simulink model "signal_simulation_test"  (R2013a)
settings: Solver=ode3  StartTime=0.0  StopTime=5  FixedStep=0.001  RelTol=1e-3
undefined symbols (not defined in the file or in its folder): sigbuilder_block
settings Model: Creator=Matthias  LastModifiedBy=Matthias

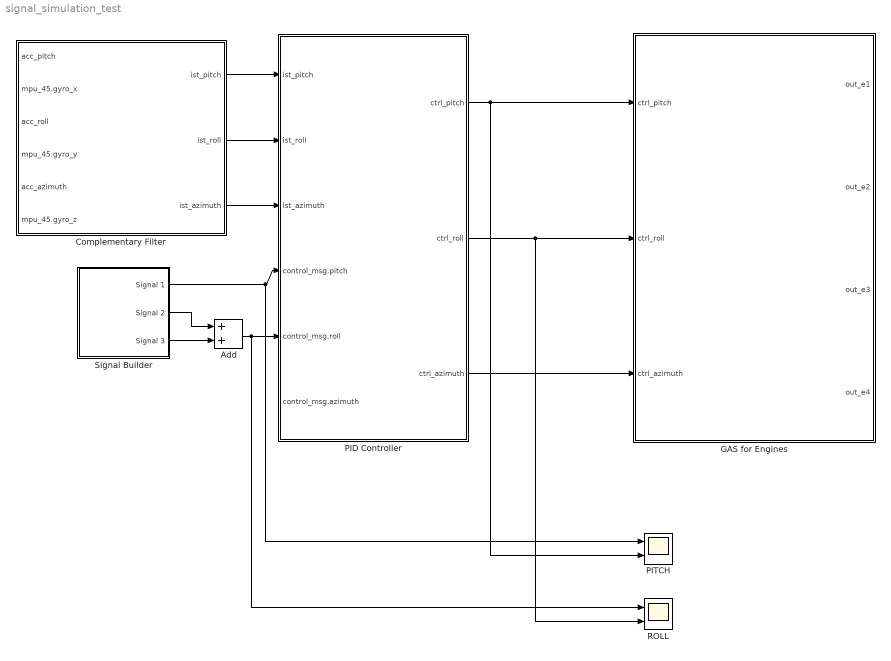
== system signal_simulation_test ==
  Add : Sum
  Complementary Filter : Subsystem
  GAS for Engines : Subsystem
  PID Controller : Subsystem
  PITCH : Scope  NumInputPorts=2
      settings: YMin=-5~-5  YMax=5~5
  ROLL : Scope  NumInputPorts=2
      settings: YMin=-5~-5  YMax=5~5
  Signal Builder : Subsystem  Tag=STV Subsys  LoadFcn=sigbuilder_block('load');  StartFcn=sigbuilder_block('start');  StopFcn=sigbuilder_block('stop');  ClipboardFcn=sigbuilder_block('clipboard');  mask(Sigbuilder block){}
      mask help: Simulink:masks:SigbuilderBlock_MD
      mask init:
      | if ~strcmp(get_param(bdroot(gcbh),'SimulationStatus'),'stopped') tuvar = sigbuilder_block('maskInit'); end
      settings: CopyFcn=sigbuilder_block('copy');  DeleteFcn=sigbuilder_block('delete');  ModelCloseFcn=sigbuilder_block('modelClose');  PreSaveFcn=sigbuilder_block('preSave');  PauseFcn=sigbuilder_block('pause');  ContinueFcn=sigbuilder_block('continue');  NameChangeFcn=sigbuilder_block('namechange');  OpenFcn=sigbuilder_block('open',[437.25 118.5 550.5 394.5 ]);  CloseFcn=sigbuilder_block('close');
      mask Display: plot(0, 0, 100, 100,[2, 2, 32, 32, 2], [68, 8, 8, 68, 68],[32, 2], [38, 38], [32, 19, 2],[53, 60, 44], [32, 17, 17, 2],[16, 16, 31, 31]);txt = getActiveGroup(gcbh);text(2, 100, txt,'verticalAlignment', 'top');
  wires:
  Complementary Filter/1(ist_pitch) -> PID Controller/1(ist_pitch)
  Complementary Filter/2(ist_roll) -> PID Controller/2(ist_roll)
  Complementary Filter/3(ist_azimuth) -> PID Controller/3(ist_azimuth)
  PID Controller/1(ctrl_pitch) -> PITCH/2, GAS for Engines/1(ctrl_pitch)
  PID Controller/2(ctrl_roll) -> ROLL/2, GAS for Engines/2(ctrl_roll)
  PID Controller/3(ctrl_azimuth) -> GAS for Engines/3(ctrl_azimuth)
  Signal Builder/1(Signal 1) -> PITCH/1, PID Controller/4(control_msg.pitch)
  Signal Builder/2(Signal 2) -> Add/1
  Add/1 -> ROLL/1, PID Controller/5(control_msg.roll)
  Signal Builder/3(Signal 3) -> Add/2

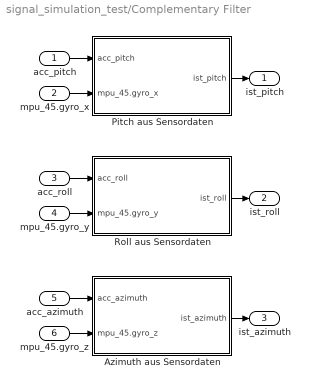
== system signal_simulation_test/Complementary Filter ==
  acc_pitch : Inport
  mpu_45.gyro_x : Inport  Port=2
  acc_roll : Inport  Port=3
  mpu_45.gyro_y : Inport  Port=4
  acc_azimuth : Inport  Port=5
  mpu_45.gyro_z : Inport  Port=6
  Azimuth aus Sensordaten : Subsystem
  Pitch aus Sensordaten : Subsystem
  Roll aus Sensordaten : Subsystem
  ist_pitch : Outport
  ist_roll : Outport  Port=2
  ist_azimuth : Outport  Port=3
  wires:
  acc_pitch/1 -> Pitch aus Sensordaten/1(acc_pitch)
  mpu_45.gyro_x/1 -> Pitch aus Sensordaten/2(mpu_45.gyro_x)
  Roll aus Sensordaten/1(ist_roll) -> ist_roll/1
  Azimuth aus Sensordaten/1(ist_azimuth) -> ist_azimuth/1
  Pitch aus Sensordaten/1(ist_pitch) -> ist_pitch/1
  mpu_45.gyro_y/1 -> Roll aus Sensordaten/2(mpu_45.gyro_y)
  acc_roll/1 -> Roll aus Sensordaten/1(acc_roll)
  mpu_45.gyro_z/1 -> Azimuth aus Sensordaten/2(mpu_45.gyro_z)
  acc_azimuth/1 -> Azimuth aus Sensordaten/1(acc_azimuth)

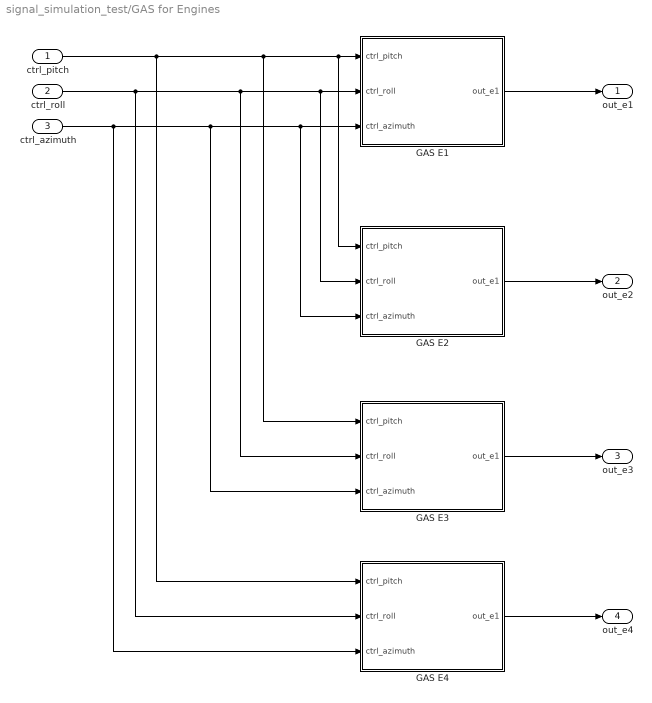
== system signal_simulation_test/GAS for Engines ==
  ctrl_pitch : Inport
  ctrl_roll : Inport  Port=2
  ctrl_azimuth : Inport  Port=3
  GAS E1 : Subsystem
  GAS E2 : Subsystem
  GAS E3 : Subsystem
  GAS E4 : Subsystem
  out_e1 : Outport
  out_e2 : Outport  Port=2
  out_e3 : Outport  Port=3
  out_e4 : Outport  Port=4
  wires:
  ctrl_pitch/1 -> GAS E2/1(ctrl_pitch), GAS E1/1(ctrl_pitch), GAS E3/1(ctrl_pitch), GAS E4/1(ctrl_pitch)
  GAS E1/1(out_e1) -> out_e1/1
  GAS E2/1(out_e1) -> out_e2/1
  ctrl_roll/1 -> GAS E4/2(ctrl_roll), GAS E1/2(ctrl_roll), GAS E2/2(ctrl_roll), GAS E3/2(ctrl_roll)
  GAS E3/1(out_e1) -> out_e3/1
  ctrl_azimuth/1 -> GAS E4/3(ctrl_azimuth), GAS E1/3(ctrl_azimuth), GAS E2/3(ctrl_azimuth), GAS E3/3(ctrl_azimuth)
  GAS E4/1(out_e1) -> out_e4/1

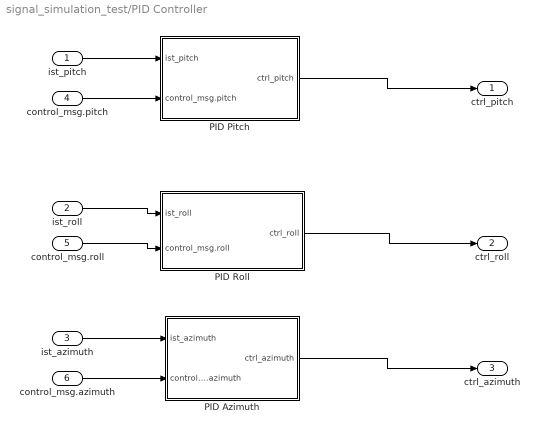
== system signal_simulation_test/PID Controller ==
  ist_pitch : Inport
  ist_roll : Inport  Port=2
  ist_azimuth : Inport  Port=3
  control_msg.pitch : Inport  Port=4
  control_msg.roll : Inport  Port=5
  control_msg.azimuth : Inport  Port=6
  PID Azimuth : Subsystem
  PID Pitch : Subsystem
  PID Roll : Subsystem
  ctrl_pitch : Outport
  ctrl_roll : Outport  Port=2
  ctrl_azimuth : Outport  Port=3
  wires:
  ist_pitch/1 -> PID Pitch/1(ist_pitch)
  control_msg.pitch/1 -> PID Pitch/2(control_msg.pitch)
  ist_azimuth/1 -> PID Azimuth/1(ist_azimuth)
  control_msg.azimuth/1 -> PID Azimuth/2(control_msg.azimuth)
  ist_roll/1 -> PID Roll/1(ist_roll)
  control_msg.roll/1 -> PID Roll/2(control_msg.roll)
  PID Pitch/1(ctrl_pitch) -> ctrl_pitch/1
  PID Roll/1(ctrl_roll) -> ctrl_roll/1
  PID Azimuth/1(ctrl_azimuth) -> ctrl_azimuth/1

== system signal_simulation_test/Signal Builder ==
  Demux : Demux  Tag=STV Demux  Outputs=3
  FromWs : FromWorkspace  Tag=STV FromWs  VariableName=tuvar  SampleTime=0
      SigBuilderData=|
      | common.afterFinalStr = 'Extrapolate'
      | common.sampleTime = 0
      | dataSet.timeRange = [0 10]
      | dataSet.name = 'Group 1'
      | sbobj.Groups.Name = 'Group 1'
      | sbobj.Groups.Signals(1).Name = 'Signal 1'
      | sbobj.Groups.Signals(1).XData = [0 1.02 1.02 3 3 10]
      | sbobj.Groups.Signals(1).YData = [0 0 1 1 0 0]
      | sbobj.Groups.Signals(2).Name = 'Signal 2'
      | sbobj.Groups.Signals(2).XData = [0 3.98 3.98 5.98 5.98 10]
      | sbobj.Groups.Signals(2).YData = [0 0 1 1 0 0]
      | sbobj.Groups.Signals(3).Name = 'Signal 3'
      | sbobj.Groups.Signals(3).XData = [0 7 7 7.96 7.96 10]
      | sbobj.Groups.Signals(3).YData = [0 0 -1.04 -1.04 0 0]
  Signal 1 : Outport  Tag=STV Outport
  Signal 2 : Outport  Tag=STV Outport  Port=2
  Signal 3 : Outport  Tag=STV Outport  Port=3
  wires:
  Demux/1 -> Signal 1/1
  FromWs/1 -> Demux/1
  Demux/2 -> Signal 2/1
  Demux/3 -> Signal 3/1

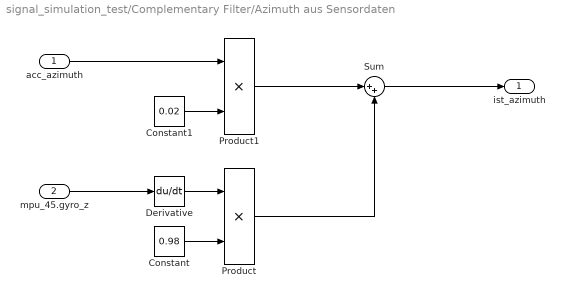
== system signal_simulation_test/Complementary Filter/Azimuth aus Sensordaten ==
  acc_azimuth : Inport
  mpu_45.gyro_z : Inport  Port=2
  Constant : Constant  Value=0.98
  Constant1 : Constant  Value=0.02
  Derivative : Derivative
  Product : Product
  Product1 : Product
  Sum : Sum  Inputs=|++
  ist_azimuth : Outport
  wires:
  mpu_45.gyro_z/1 -> Derivative/1
  Derivative/1 -> Product/1
  Constant/1 -> Product/2
  Constant1/1 -> Product1/2
  acc_azimuth/1 -> Product1/1
  Product1/1 -> Sum/1
  Product/1 -> Sum/2
  Sum/1 -> ist_azimuth/1

== system signal_simulation_test/Complementary Filter/Pitch aus Sensordaten ==
  acc_pitch : Inport
  mpu_45.gyro_x : Inport  Port=2
  Constant : Constant  Value=0.98
  Constant1 : Constant  Value=0.02
  Derivative : Derivative
  Product : Product
  Product1 : Product
  Sum : Sum  Inputs=|++
  ist_pitch : Outport
  wires:
  mpu_45.gyro_x/1 -> Derivative/1
  Derivative/1 -> Product/1
  Constant/1 -> Product/2
  Constant1/1 -> Product1/2
  acc_pitch/1 -> Product1/1
  Product1/1 -> Sum/1
  Product/1 -> Sum/2
  Sum/1 -> ist_pitch/1

== system signal_simulation_test/Complementary Filter/Roll aus Sensordaten ==
  acc_roll : Inport
  mpu_45.gyro_y : Inport  Port=2
  Constant : Constant  Value=0.98
  Constant1 : Constant  Value=0.02
  Derivative : Derivative
  Product : Product
  Product1 : Product
  Sum : Sum  Inputs=|++
  ist_roll : Outport
  wires:
  mpu_45.gyro_y/1 -> Derivative/1
  Derivative/1 -> Product/1
  Constant/1 -> Product/2
  Constant1/1 -> Product1/2
  acc_roll/1 -> Product1/1
  Product1/1 -> Sum/1
  Product/1 -> Sum/2
  Sum/1 -> ist_roll/1

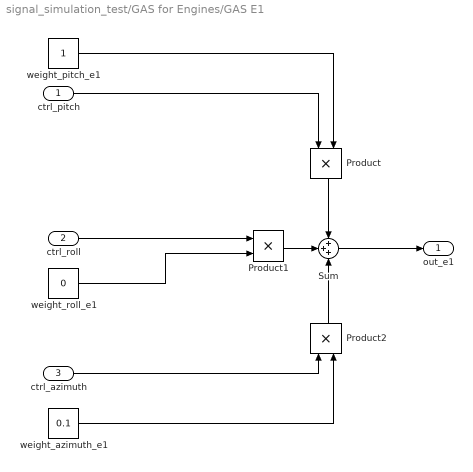
== system signal_simulation_test/GAS for Engines/GAS E1 ==
  ctrl_pitch : Inport
  ctrl_roll : Inport  Port=2
  ctrl_azimuth : Inport  Port=3
  Product : Product
  Product1 : Product
  Product2 : Product
  Sum : Sum  Inputs=+++
  weight_azimuth_e1 : Constant  Value=0.1
  weight_pitch_e1 : Constant
  weight_roll_e1 : Constant  Value=0
  out_e1 : Outport
  wires:
  Product/1 -> Sum/1
  Sum/1 -> out_e1/1
  Product1/1 -> Sum/2
  Product2/1 -> Sum/3
  ctrl_roll/1 -> Product1/1
  ctrl_pitch/1 -> Product/1
  ctrl_azimuth/1 -> Product2/1
  weight_roll_e1/1 -> Product1/2
  weight_pitch_e1/1 -> Product/2
  weight_azimuth_e1/1 -> Product2/2

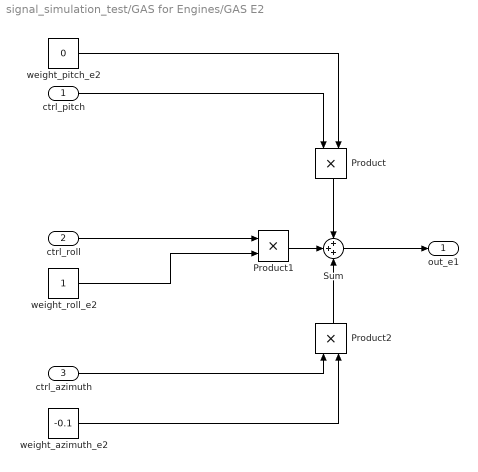
== system signal_simulation_test/GAS for Engines/GAS E2 ==
  ctrl_pitch : Inport
  ctrl_roll : Inport  Port=2
  ctrl_azimuth : Inport  Port=3
  Product : Product
  Product1 : Product
  Product2 : Product
  Sum : Sum  Inputs=+++
  weight_azimuth_e2 : Constant  Value=-0.1
  weight_pitch_e2 : Constant  Value=0
  weight_roll_e2 : Constant
  out_e1 : Outport
  wires:
  Product/1 -> Sum/1
  Sum/1 -> out_e1/1
  Product1/1 -> Sum/2
  Product2/1 -> Sum/3
  ctrl_roll/1 -> Product1/1
  ctrl_pitch/1 -> Product/1
  ctrl_azimuth/1 -> Product2/1
  weight_roll_e2/1 -> Product1/2
  weight_pitch_e2/1 -> Product/2
  weight_azimuth_e2/1 -> Product2/2

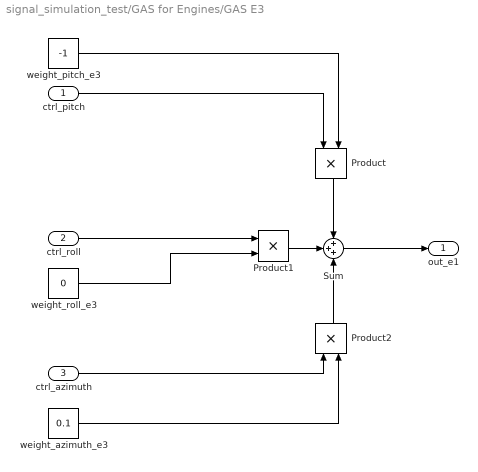
== system signal_simulation_test/GAS for Engines/GAS E3 ==
  ctrl_pitch : Inport
  ctrl_roll : Inport  Port=2
  ctrl_azimuth : Inport  Port=3
  Product : Product
  Product1 : Product
  Product2 : Product
  Sum : Sum  Inputs=+++
  weight_azimuth_e3 : Constant  Value=0.1
  weight_pitch_e3 : Constant  Value=-1
  weight_roll_e3 : Constant  Value=0
  out_e1 : Outport
  wires:
  Product/1 -> Sum/1
  Sum/1 -> out_e1/1
  Product1/1 -> Sum/2
  Product2/1 -> Sum/3
  ctrl_roll/1 -> Product1/1
  ctrl_pitch/1 -> Product/1
  ctrl_azimuth/1 -> Product2/1
  weight_roll_e3/1 -> Product1/2
  weight_pitch_e3/1 -> Product/2
  weight_azimuth_e3/1 -> Product2/2

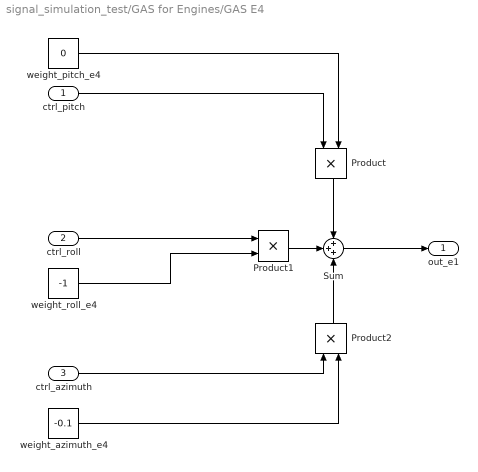
== system signal_simulation_test/GAS for Engines/GAS E4 ==
  ctrl_pitch : Inport
  ctrl_roll : Inport  Port=2
  ctrl_azimuth : Inport  Port=3
  Product : Product
  Product1 : Product
  Product2 : Product
  Sum : Sum  Inputs=+++
  weight_azimuth_e4 : Constant  Value=-0.1
  weight_pitch_e4 : Constant  Value=0
  weight_roll_e4 : Constant  Value=-1
  out_e1 : Outport
  wires:
  Product/1 -> Sum/1
  Sum/1 -> out_e1/1
  Product1/1 -> Sum/2
  Product2/1 -> Sum/3
  ctrl_roll/1 -> Product1/1
  ctrl_pitch/1 -> Product/1
  ctrl_azimuth/1 -> Product2/1
  weight_roll_e4/1 -> Product1/2
  weight_pitch_e4/1 -> Product/2
  weight_azimuth_e4/1 -> Product2/2

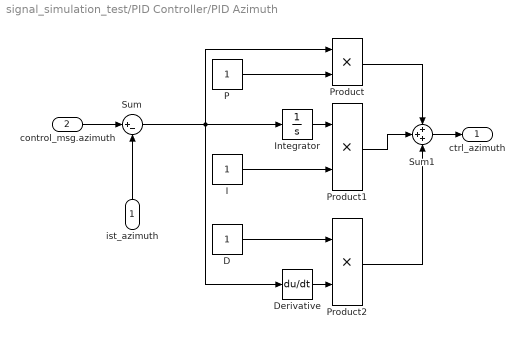
== system signal_simulation_test/PID Controller/PID Azimuth ==
  ist_azimuth : Inport
  control_msg.azimuth : Inport  Port=2
  D : Constant
  Derivative : Derivative
  I : Constant
  Integrator : Integrator
  P : Constant
  Product : Product
  Product1 : Product
  Product2 : Product
  Sum : Sum  Inputs=|+-
  Sum1 : Sum  Inputs=+++
  ctrl_azimuth : Outport
  wires:
  ist_azimuth/1 -> Sum/2
  control_msg.azimuth/1 -> Sum/1
  Sum1/1 -> ctrl_azimuth/1
  Sum/1 -> Derivative/1, Product/1, Integrator/1
  P/1 -> Product/2
  Product/1 -> Sum1/1
  Product1/1 -> Sum1/2
  Integrator/1 -> Product1/1
  I/1 -> Product1/2
  Product2/1 -> Sum1/3
  Derivative/1 -> Product2/2
  D/1 -> Product2/1

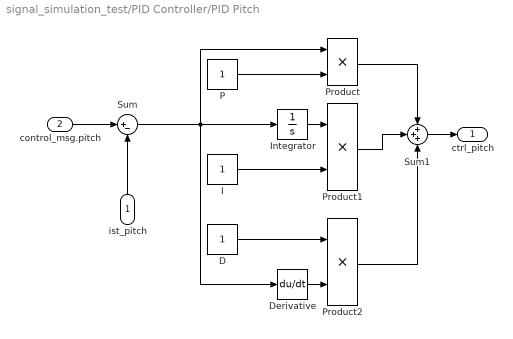
== system signal_simulation_test/PID Controller/PID Pitch ==
  ist_pitch : Inport
  control_msg.pitch : Inport  Port=2
  D : Constant
  Derivative : Derivative
  I : Constant
  Integrator : Integrator
  P : Constant
  Product : Product
  Product1 : Product
  Product2 : Product
  Sum : Sum  Inputs=|+-
  Sum1 : Sum  Inputs=+++
  ctrl_pitch : Outport
  wires:
  ist_pitch/1 -> Sum/2
  control_msg.pitch/1 -> Sum/1
  Sum1/1 -> ctrl_pitch/1
  Sum/1 -> Derivative/1, Product/1, Integrator/1
  P/1 -> Product/2
  Product/1 -> Sum1/1
  Product1/1 -> Sum1/2
  Integrator/1 -> Product1/1
  I/1 -> Product1/2
  Product2/1 -> Sum1/3
  Derivative/1 -> Product2/2
  D/1 -> Product2/1

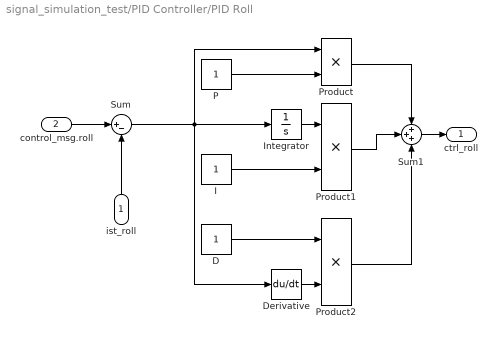
== system signal_simulation_test/PID Controller/PID Roll ==
  ist_roll : Inport
  control_msg.roll : Inport  Port=2
  D : Constant
  Derivative : Derivative
  I : Constant
  Integrator : Integrator
  P : Constant
  Product : Product
  Product1 : Product
  Product2 : Product
  Sum : Sum  Inputs=|+-
  Sum1 : Sum  Inputs=+++
  ctrl_roll : Outport
  wires:
  ist_roll/1 -> Sum/2
  control_msg.roll/1 -> Sum/1
  Sum1/1 -> ctrl_roll/1
  Sum/1 -> Derivative/1, Product/1, Integrator/1
  P/1 -> Product/2
  Product/1 -> Sum1/1
  Product1/1 -> Sum1/2
  Integrator/1 -> Product1/1
  I/1 -> Product1/2
  Product2/1 -> Sum1/3
  Derivative/1 -> Product2/2
  D/1 -> Product2/1
